simulink model "androidSensorFilterExample"  (R2022a)
settings: Solver=ode3  StartTime=0.0  StopTime=40  RelTol=1e-3
undefined symbols (not defined in the file): fdesignblkfcn, gcbh
libraries: androidsensorlib x1, realtime_examples_misc x1
PreSaveFcn:
  | set_param(gcs, 'Location',[35 56 895 605])
settings Model: SimulationMode=external  ExtModeTrigDuration=100  Creator=The MathWorks, Inc.  LastModifiedBy=USER
settings SolverCC: AlgebraicLoopSolver=TrustRegion
settings DataIOCC: LimitDataPoints=on  SaveFormat=Array  ReturnWorkspaceOutputs=off
settings OptimizationCC: LifeSpan=1  MaxStackSize=64
settings DebuggingCC: UnderspecifiedInitializationDetection=Classic  MergeDetectMultiDrivingBlocksExec=none  ParameterPrecisionLossMsg=none  UnconnectedInputMsg=warning  UnconnectedOutputMsg=warning  UnconnectedLineMsg=warning  AllowSymbolicDim=off  SFUnexpectedBacktrackingDiag=warning  SFNoUnconditionalDefaultTransitionDiag=warning  SFExecutionAtInitializationDiag=none  SFMachineParentedDataDiag=warning  ArithmeticOperatorsInVariantConditions=warning
settings HardwareCC: ProdBitPerPointer=32  ProdLargestAtomicInteger=Long  ProdLargestAtomicFloat=Double  ProdWordSize=32  ProdHWDeviceType=ARM Compatible->ARM Cortex  TargetLargestAtomicInteger=Long  TargetLargestAtomicFloat=Double  TargetEndianess=LittleEndian  TargetHWDeviceType=ARM Compatible->ARM Cortex  UseEmbeddedCoderFeatures=off  UseSimulinkCoderFeatures=off
settings ModelReferenceCC: PropagateSignalLabelsOutOfModel=off
settings SFSimCC: SimUseLocalCustomCode=off  CustomCodeUndefinedFunction=UseInterfaceOnly
settings RTWCC: SystemTargetFile=ert.tlc  HardwareBoard=Android Device  TemplateMakefile=ert_default_tmf  GenerateReport=on  RTWVerbose=off  RTWUseLocalCustomCode=off  Toolchain=Android SDK/NDK Tools  LaunchReport=on
settings CodeAppCC: ForceParamTrailComments=on  OperatorAnnotations=on  StateflowObjectComments=on  MATLABSourceComments=on
settings ERTTargetCC: MultiwordLength=2048  ERTCustomFileBanners=off  SupportContinuousTime=on  SupportNonInlinedSFcns=on  RemoveResetFunc=off  ModelStepFunctionPrototypeControlCompliant=off
settings ConfigComp: CovMetricSettings=dw  CovSaveCumulativeToWorkspaceVar=on  CovSaveSingleToWorkspaceVar=on  CovExternalEMLEnable=off  CovSFcnEnable=off

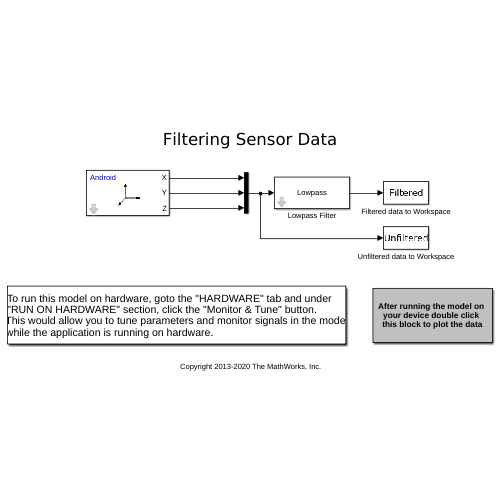
[thumbnail: Simulink's stored preview of the top-level diagram]
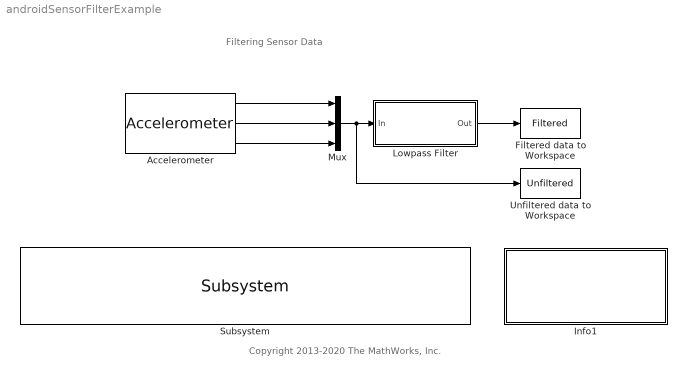
== system androidSensorFilterExample ==
  note: Copyright 2013-2020 The MathWorks, Inc.
  note: Filtering Sensor Data
  Accelerometer : androidsensorlib/Accelerometer  OutputVector=off  SampleTime=0.1  BlockPlatform=Android
      settings: SourceProductBaseCode=ANDROID
  Filtered data to Workspace : ToWorkspace  VariableName=Filtered  SaveFormat=Structure With Time  SampleTime=-1
  Info1 : Subsystem  Description=Descibes demo and operating procedure.
      settings: OpenFcn=android_plotsensordata(bdroot);
      mask Display: fprintf('After running the model on \nyour device double click \nthis block to plot the data')
  Lowpass Filter : Subsystem  DialogController=fdesignblkfcn  InitFcn=fdesignblkfcn(gcbh, {'InitFcn'});  mask(Lowpass Filter){}
      mask help: Design a lowpass filter
      settings: CopyFcn=fdesignblkfcn(gcbh, {'CopyFcn'});
      mask Help: helpview(mapfilelocation('dsp'), 'dsplowpassfilter');
      mask Display: disp('Lowpass')
  Mux : Mux  Inputs=3
  Subsystem : realtime_examples_misc/Subsystem  SystemSampleTime=-1  VariantActivationTime=update diagram  Latency=0  AutoFrameSizeCalculation=off
      settings: SourceProductBaseCode=SL
  Unfiltered data to Workspace : ToWorkspace  VariableName=Unfiltered  SaveFormat=Structure With Time  SampleTime=-1
  wires:
  Mux/1 -> Lowpass Filter/1(In), Unfiltered data to Workspace/1
  Accelerometer/3 -> Mux/3
  Accelerometer/1 -> Mux/1
  Accelerometer/2 -> Mux/2
  Lowpass Filter/1(Out) -> Filtered data to Workspace/1

== system androidSensorFilterExample/Info1 ==

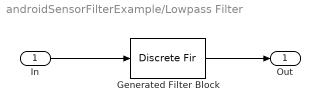
== system androidSensorFilterExample/Lowpass Filter ==
  In : Inport
  Generated Filter Block : DiscreteFir  Tag=BlockMethodSubSystem  Coefficients=[-0.00096423888646545363 -0.0014108375177254192 -0.0022412546182366496 -0.003178898224895416 -0.0041019075331767971 -0.004853293298414366 -0.0052505134309028777 -0.0051161236392097253 -0.0043118443099008398 -0.0027731899953295129 -0.00053947529829025858 0.0022274442736046783 0.005240855952785054 0.0081088553185423625 0.010376636014246541 0.011586749865337493 0.01135201960547421 0.009431830651362931 0.00579898459885363 0.00068561216866704143 -0.0054023448939036628 -0.011709241472406441 -0.017293108020851169 -0.021124248149764359 -0.022209696784074723 -0.019728125995165345 -0.013156997241206066 -0.0023735292112024063 0.012286828258260166 0.03002553370523859 0.049634115918957472 0.069602197336891408 0.08826934096899236 0.10400284916091337 0.1153793066919762 0.12134681081050722 0.12134681081050722 0.1153793066919762 0.10400284916091337 0.08826934096899236 0.069602197336891408 0.049634115918957472 0.03002553370523859 0.012286828258260166 -0.0023735292112024063 -0.013156997241206066 -0.019728125995165345 -0.022209696784074723 -0.021124248149764359 -0.017293108020851169 -0.011709241472406441 -0.0054023448939036628 0.00068561216866704143 0.00579898459885363 0.009431830651362931 0.01135201960547421 0.011586749865337493 0.010376636014246541 0.0081088553185423625 0.005240855952785054 0.0022274442736046783 -0.00053947529829025858 -0.0027731899953295129 -0.0043118443099008398 -0.0051161236392097253 -0.0052505134309028777 -0.004853293298414366 -0.0041019075331767971 -0.003178898224895416 -0.0022412546182366496 -0.0014108375177254192 -0.00096423888646545363]
  Out : Outport
  wires:
  Generated Filter Block/1 -> Out/1
  In/1 -> Generated Filter Block/1
